simulink model "Practica"  (R2021a)
settings: Solver=FixedStepAuto  StartTime=0.0  StopTime=50.0  FixedStep=0.01  RelTol=1e-3
undefined symbols (not defined in the file or in its folder): b, k, m
libraries: simulink x1
settings Model: Creator=e.delpico.2020  LastModifiedBy=e.delpico.2020

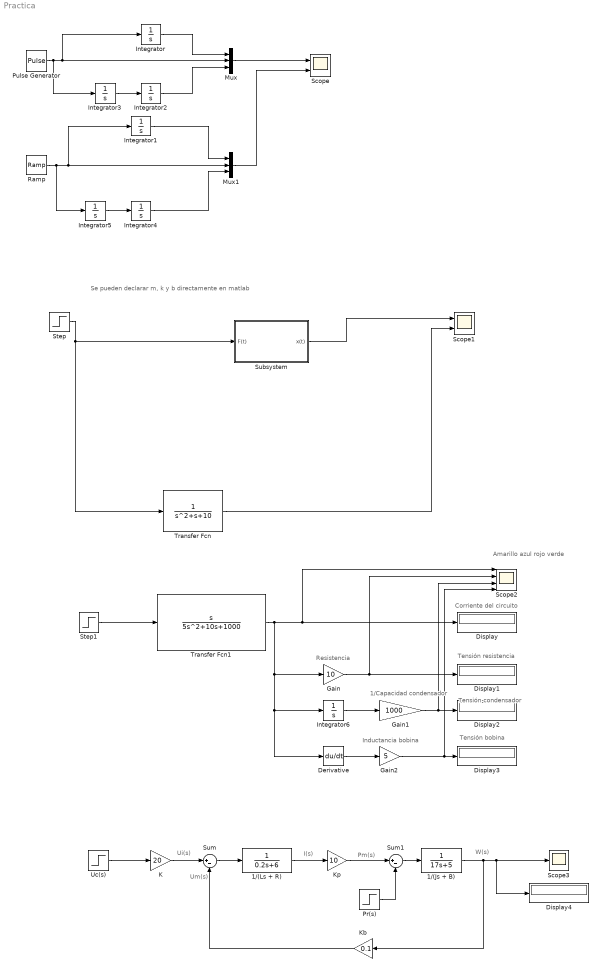
== system Practica ==
  note: W(s)
  note: Pm(s)
  note: Um(s)
  note: I(s)
  note: Ui(s)
  note: Amarillo azul rojo verde
  note: Tensión bobina
  note: Tensión condensador
  note: Tensión resistencia
  note: Corriente del circuito
  note: Inductancia bobina
  note: 1/Capacidad condensador
  note: Resistencia
  note: Se pueden declarar m, k y b directamente en matlab
  1/(Js + B) : TransferFcn  Denominator=[17 5]
  1/(Ls + R) : TransferFcn  Denominator=[0.2 6]
  Derivative : Derivative
  Display{,1..4} (5 alike) : Display
  Gain : Gain  Gain=10
  Gain1 : Gain  Gain=1000
  Gain2 : Gain  Gain=5
  Integrator{,1..6} (7 alike) : Integrator
  K : Gain  Gain=20
  Kb : Gain  Gain=0.1
  Kp : Gain  Gain=10
  Mux : Mux  Inputs=3
  Mux1 : Mux  Inputs=3
  Pr(s) : Step  Time=20  After=120  SampleTime=0
  Pulse Generator : DiscretePulseGenerator  PulseType=Time based  Period=10  PulseWidth=5
  Ramp : simulink/Sources/Ramp  slope=1  start=0  InitialOutput=0
  Scope : Scope  NumInputPorts=2
  Scope1 : Scope  NumInputPorts=2
  Scope2 : Scope  NumInputPorts=4
  Scope3 : Scope
  Step : Step  Time=0  SampleTime=0
  Step1 : Step  Time=0  SampleTime=0
  Subsystem : Subsystem
  Sum : Sum  Inputs=|+-
  Sum1 : Sum  Inputs=|+-
  Transfer Fcn : TransferFcn  Denominator=[1 1 10]
  Transfer Fcn1 : TransferFcn  Numerator=[1 0]  Denominator=[5 10 1000]
  Uc(s) : Step  Time=0  After=20  SampleTime=0
  wires:
  Mux/1 -> Scope/1
  Pulse Generator/1 -> Mux/2, Integrator/1, Integrator3/1
  Integrator1/1 -> Mux1/1
  Mux1/1 -> Scope/2
  Integrator/1 -> Mux/1
  Integrator2/1 -> Mux/3
  Integrator3/1 -> Integrator2/1
  Integrator4/1 -> Mux1/3
  Integrator5/1 -> Integrator4/1
  Ramp/1 -> Integrator5/1, Integrator1/1, Mux1/2
  Step/1 -> Subsystem/1(F(t)), Transfer Fcn/1
  Transfer Fcn/1 -> Scope1/2
  Subsystem/1(x(t)) -> Scope1/1
  Step1/1 -> Transfer Fcn1/1
  Transfer Fcn1/1 -> Gain/1, Derivative/1, Integrator6/1, Scope2/1, Display/1
  Gain/1 -> Scope2/2, Display1/1
  Integrator6/1 -> Gain1/1
  Gain1/1 -> Scope2/3, Display2/1
  Gain2/1 -> Scope2/4, Display3/1
  Derivative/1 -> Gain2/1
  Uc(s)/1 -> K/1
  Kb/1 -> Sum/2
  Sum/1 -> 1/(Ls + R)/1
  1/(Ls + R)/1 -> Kp/1
  K/1 -> Sum/1
  Kp/1 -> Sum1/1
  Sum1/1 -> 1/(Js + B)/1
  Pr(s)/1 -> Sum1/2
  1/(Js + B)/1 -> Kb/1, Display4/1, Scope3/1

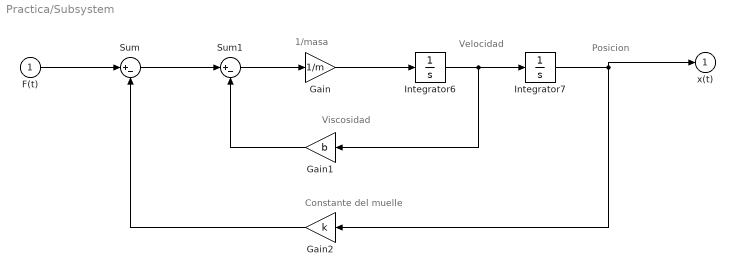
== system Practica/Subsystem ==
  note: 1/masa
  note: Velocidad
  note: Posicion
  note: Viscosidad
  note: Constante del muelle
  F(t) : Inport
  Gain : Gain  Gain=1/m
  Gain1 : Gain  Gain=b
  Gain2 : Gain  Gain=k
  Integrator6 : Integrator
  Integrator7 : Integrator
  Sum : Sum  Inputs=|+-
  Sum1 : Sum  Inputs=|+-
  x(t) : Outport
  wires:
  Gain1/1 -> Sum1/2
  Sum/1 -> Sum1/1
  Integrator7/1 -> x(t)/1, Gain2/1
  Gain/1 -> Integrator6/1
  Integrator6/1 -> Gain1/1, Integrator7/1
  F(t)/1 -> Sum/1
  Sum1/1 -> Gain/1
  Gain2/1 -> Sum/2
